simulink model "powerdistributionDC2AC"  (R2017a)
settings: Solver=VariableStepAuto  StartTime=0.0  StopTime=0.1  RelTol=1e-3
libraries: powerlib x13, simulink x1
settings Model: Creator=Nihal  LastModifiedBy=Nihal
settings DataIOCC: ReturnWorkspaceOutputs=on
settings SFSimCC: SimUseLocalCustomCode=on
settings RTWCC: RTWUseLocalCustomCode=on

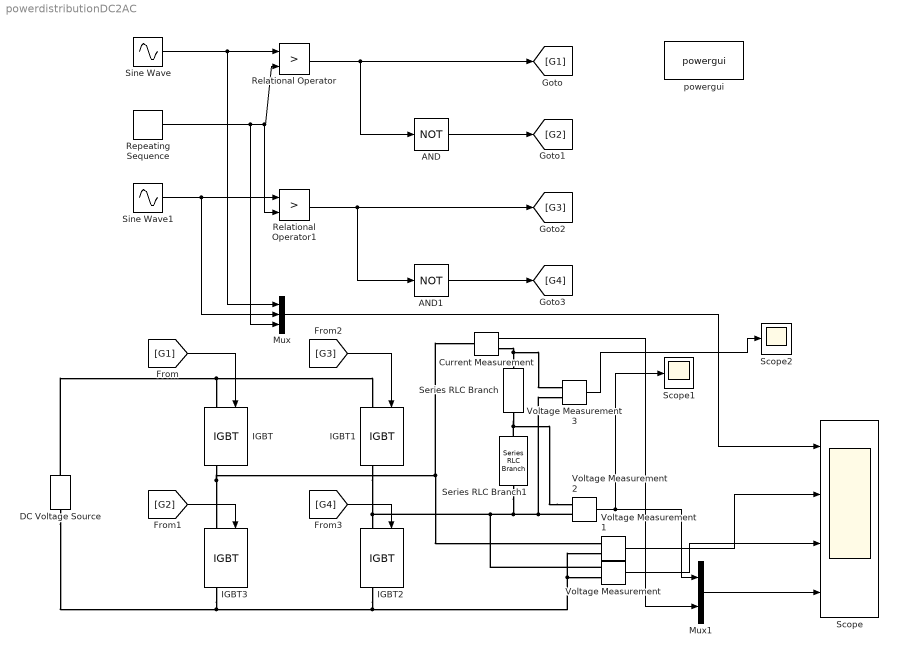
== system powerdistributionDC2AC ==
  AND : Logic  Operator=NOT  IconShape=distinctive  AllPortsSameDT=off  OutDataTypeStr=boolean
  AND1 : Logic  Operator=NOT  IconShape=distinctive  AllPortsSameDT=off  OutDataTypeStr=boolean
  Current Measurement : powerlib/Measurements/Current Measurement  PhasorSimulation=off  OutputType=Complex  PSBequivalent=0
      settings: SourceProductName=Simscape Electrical
  DC Voltage Source : powerlib/Electrical Sources/DC Voltage Source  Amplitude=20  Measurements=None
      settings: SourceProductName=Simscape Electrical
  IGBT{,1..3} (4 alike) : powerlib/Power Electronics/IGBT  Ron=0.001  Lon=0  Vf=1  Tf=1e-6  Tt=2e-6  IC=0  Rs=1e5  Cs=inf  Measurements=on
      settings: SourceProductName=Simscape Electrical
  Mux : Mux  Inputs=3
  Mux1 : Mux  Inputs=2
  Relational Operator : RelationalOperator  Operator=>  OutDataTypeStr=boolean  RndMeth=Simplest
  Relational Operator1 : RelationalOperator  Operator=>  OutDataTypeStr=boolean  RndMeth=Simplest
  Repeating Sequence : simulink/Sources/Repeating Sequence  rep_seq_t=[0 1/(4*12*50) 3/(4*12*50) 1/(12*50)]  rep_seq_y=[0 -1 1 0]
  Scope : Scope  NumInputPorts=4
  Scope1 : Scope
  Scope2 : Scope
  Series RLC Branch : powerlib/Elements/Series RLC Branch  LConnTagsString=__new0  RConnTagsString=__new0  BranchType=R  Resistance=1000  Inductance=1e-3  SetiL0=off  InitialCurrent=0  Capacitance=1e-6  Setx0=off  InitialVoltage=0  Measurements=None
      settings: SourceProductName=Simscape Electrical
  Series RLC Branch1 : powerlib/Elements/Series RLC Branch  LConnTagsString=__new0  RConnTagsString=__new0  BranchType=C  Resistance=1  Inductance=1e-3  SetiL0=off  InitialCurrent=0  Capacitance=4.00e-8  Setx0=off  InitialVoltage=0  Measurements=None
      settings: SourceProductName=Simscape Electrical
  Sine Wave : Sin  Amplitude=0.8  Frequency=100*pi  SampleTime=0
  Sine Wave1 : Sin  Amplitude=0.8  Frequency=100*pi  Phase=pi  SampleTime=0
  Voltage Measurement{,1..3} (4 alike) : powerlib/Measurements/Voltage Measurement  PhasorSimulation=off  OutputType=Complex  PSBequivalent=0
      settings: SourceProductName=Simscape Electrical
  powergui : powerlib/powergui  Priority=1  SimulationMode=Discrete  SampleTime=1e-05  frequency=60  Iterations=50  frequencyindice=0  Pbase=100e6  ErrMax=1e-4  UnitsV=kV  UnitsW=MW  buscounter=0  FunctionMessages=off  echomessages=off  EnableUseOfTLC=off  CurrentSourceSwitches=off  DisableSnubberDevices=off  DisableRonSwitches=off  DisableVfSwitches=off  DisplayEquations=off  AutomaticDiscreteSolvers=off  SolverType=Tustin/Backward Euler (TBE)  Interpol=off  ExternalGateDelay=off  methode=off  Ts=100  x0status=blocks  SPID=on  SwTol=0  HookPort=off  NonlinearTolerance=1e-4  nMaxIteration=100  ContinueOnMaxIteration=off  RestoreLinks=warning  ResistiveCurrentMeasurement=off  Frange=[0:2:500]  Ylog=off  Xlog=on  ShowGrid=off  save=off  variable=ZData  structure=0  ZoomFFT=off  StartTime=0.0  cycles=1  DisplayStyle=1  fundamental=60  FreqAxis=off  MaxFrequency=1000  frequencyindicesteady=1  RmsSteady=1  display=off
      settings: SourceProductName=Simscape Electrical
  wires:
  Repeating Sequence/1 -> Relational Operator1/2, Relational Operator/2, Mux/3
  Sine Wave1/1 -> Relational Operator1/1, Mux/2
  Sine Wave/1 -> Relational Operator/1, Mux/1
  Relational Operator1/1 -> AND1/1, [G3]
  AND1/1 -> [G4]
  Relational Operator/1 -> AND/1, [G1]
  AND/1 -> [G2]
  [G2] -> IGBT3/1
  [G4] -> IGBT2/1
  [G3] -> IGBT1/1
  [G1] -> IGBT/1
  Mux/1 -> Scope/1
  Mux1/1 -> Scope/4
  Voltage Measurement/1 -> Scope/3
  Voltage Measurement1/1 -> Scope/2
  Voltage Measurement2/1 -> Scope1/1, Mux1/1
  Current Measurement/1 -> Mux1/2
  Voltage Measurement3/1 -> Scope2/1
  connections:
  DC Voltage Source/RConn1 -- IGBT/LConn1 -- IGBT1/LConn1
  IGBT/RConn1 -- IGBT3/LConn1 -- Voltage Measurement1/LConn1 -- Current Measurement/LConn1
  DC Voltage Source/LConn1 -- IGBT3/RConn1 -- Voltage Measurement1/LConn2 -- Voltage Measurement/LConn2 -- IGBT2/RConn1
  Current Measurement/RConn1 -- Voltage Measurement3/LConn1 -- Series RLC Branch/RConn1
  Voltage Measurement2/LConn1 -- Series RLC Branch1/LConn1 -- Series RLC Branch/LConn1
  Series RLC Branch1/RConn1 -- Voltage Measurement2/LConn2 -- Voltage Measurement3/LConn2 -- IGBT1/RConn1 -- IGBT2/LConn1 -- Voltage Measurement/LConn1
